simulink model "admittance"  (Simulink 8.5)
settings: Solver=ode15s  SolverMode=SingleTasking  StartTime=0.0  StopTime=0.1  RelTol=1e-3  AbsTol=1e-6
libraries: powerlib x25, powerlib_extras x6
settings Model: Creator=Dr. Lotfifard  LastModifiedBy=PC  ExtModeTrigMode=oneshot  ExtModeArmWhenConnect=off
settings DataIOCC: LimitDataPoints=off
settings OptimizationCC: BlockReduction=off  BooleanDataType=off
settings DebuggingCC: SaveWithParameterizedLinksMsg=none  SignalResolutionControl=TryResolveAllWithWarning  MultiTaskDSMMsg=warning  MultiTaskCondExecSysMsg=none  FcnCallInpInsideContextMsg=UseLocalSettings  StrictBusMsg=None
settings HardwareCC: TargetUnknown=on

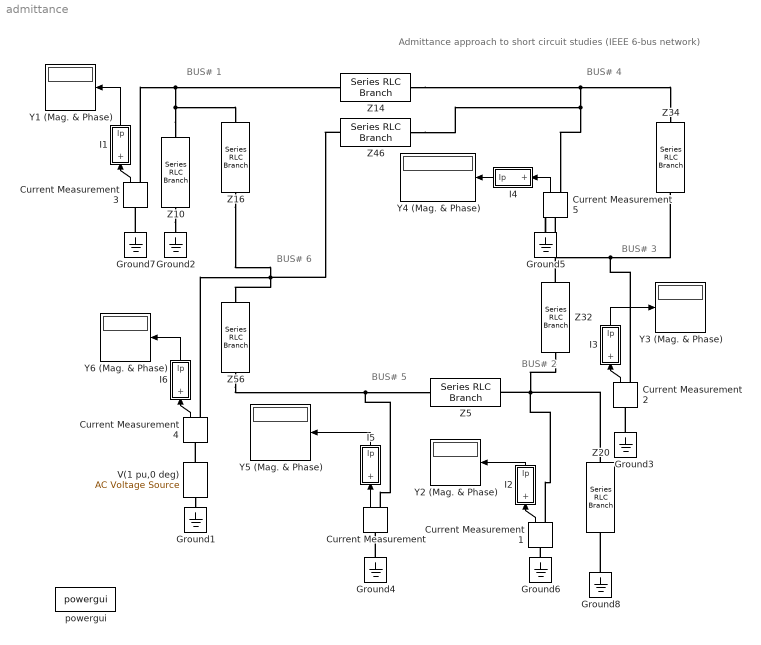
== system admittance ==
  note: Admittance approach to short circuit studies
      | (IEEE 6-bus network)
  note: BUS# 1
  note: BUS# 4
  note: BUS# 6
  note: BUS# 3
  note: BUS# 2
  note: BUS# 5
  Current Measurement{,1..5} (6 alike) : powerlib/Measurements/Current Measurement  PhasorSimulation=off  OutputType=Complex  PSBequivalent=0
  Ground{1..8} (8 alike) : powerlib/Elements/Ground  LConnTagsString=a
  I1 : Subsystem
  I2 : Subsystem
  I3 : Subsystem
  I4 : Subsystem
  I5 : Subsystem
  I6 : Subsystem
  V(1 pu,0 deg) : powerlib/Electrical Sources/AC Voltage Source  Amplitude=1  Phase=0  Frequency=60  SampleTime=0  Measurements=None
  Y1 (Mag. & Phase) : Display
  Y2 (Mag. & Phase) : Display
  Y3 (Mag. & Phase) : Display
  Y4 (Mag. & Phase) : Display
  Y5 (Mag. & Phase) : Display
  Y6 (Mag. & Phase) : Display
  Z10 : powerlib/Elements/Series RLC Branch  LConnTagsString=__new0  RConnTagsString=__new0  BranchType=RL  Resistance=0.02  Inductance=0.24/(2*pi*60)  SetiL0=off  InitialCurrent=0  Capacitance=1e-6  Setx0=off  InitialVoltage=0  Measurements=None
  Z14 : powerlib/Elements/Series RLC Branch  LConnTagsString=__new0  RConnTagsString=__new0  BranchType=RL  Resistance=0.16  Inductance=0.74/(2*pi*60)  SetiL0=off  InitialCurrent=0  Capacitance=1e-6  Setx0=off  InitialVoltage=0  Measurements=None
  Z16 : powerlib/Elements/Series RLC Branch  LConnTagsString=__new0  RConnTagsString=__new0  BranchType=RL  Resistance=0.246  Inductance=1.036/(2*pi*60)  SetiL0=off  InitialCurrent=0  Capacitance=1e-6  Setx0=off  InitialVoltage=0  Measurements=None
  Z20 : powerlib/Elements/Series RLC Branch  LConnTagsString=__new0  RConnTagsString=__new0  BranchType=RL  Resistance=0.03  Inductance=0.48/(2*pi*60)  SetiL0=off  InitialCurrent=0  Capacitance=1e-6  Setx0=off  InitialVoltage=0  Measurements=None
  Z32 : powerlib/Elements/Series RLC Branch  LConnTagsString=__new0  RConnTagsString=__new0  BranchType=RL  Resistance=1.446  Inductance=2.1/(2*pi*60)  SetiL0=off  InitialCurrent=0  Capacitance=1e-6  Setx0=off  InitialVoltage=0  Measurements=None
  Z34 : powerlib/Elements/Series RLC Branch  LConnTagsString=__new0  RConnTagsString=__new0  BranchType=RL  Resistance=0  Inductance=0.266/(2*pi*60)  SetiL0=off  InitialCurrent=0  Capacitance=1e-6  Setx0=off  InitialVoltage=0  Measurements=None
  Z46 : powerlib/Elements/Series RLC Branch  LConnTagsString=__new0  RConnTagsString=__new0  BranchType=RL  Resistance=0.194  Inductance=0.814/(2*pi*60)  SetiL0=off  InitialCurrent=0  Capacitance=1e-6  Setx0=off  InitialVoltage=0  Measurements=None
  Z5 : powerlib/Elements/Series RLC Branch  LConnTagsString=__new0  RConnTagsString=__new0  BranchType=RL  Resistance=0.564  Inductance=1.28/(2*pi*60)  SetiL0=off  InitialCurrent=0  Capacitance=1e-6  Setx0=off  InitialVoltage=0  Measurements=None
  Z56 : powerlib/Elements/Series RLC Branch  LConnTagsString=__new0  RConnTagsString=__new0  BranchType=RL  Resistance=0  Inductance=0.6/(2*pi*60)  SetiL0=off  InitialCurrent=0  Capacitance=1e-6  Setx0=off  InitialVoltage=0  Measurements=None
  powergui : powerlib/powergui  SimulationMode=Continuous  SolverType=Tustin/Backward Euler (TBE)  SampleTime=0  frequency=60  SPID=off  DisableSnubberDevices=off  DisableRonSwitches=off  DisableVfSwitches=off  SwTol=0  DisplayEquations=off  Interpol=off  methode=off  Ts=0  FunctionMessages=off  echomessages=off  HookPort=off  EnableUseOfTLC=off  x0status=blocks  frequencyindice=60  Pbase=100e6  ErrMax=1e-4  Iterations=50  UnitsV=kV  UnitsW=MW  buscounter=0  RestoreLinks=warning  ResistiveCurrentMeasurement=off  Frange=[0:2:500]  Ylog=off  Xlog=on  ShowGrid=off  save=off  variable=ZData  structure=0  ZoomFFT=on  StartTime=0.0  cycles=1  DisplayStyle=1  fundamental=60  FreqAxis=off  MaxFrequency=1000  frequencyindicesteady=1  RmsSteady=1  display=off
  wires:
  Current Measurement/1 -> I5/1(+)
  I5/1(Ip) -> Y5 (Mag. & Phase)/1
  Current Measurement1/1 -> I2/1(+)
  I2/1(Ip) -> Y2 (Mag. & Phase)/1
  Current Measurement2/1 -> I3/1(+)
  I3/1(Ip) -> Y3 (Mag. & Phase)/1
  Current Measurement3/1 -> I1/1(+)
  I1/1(Ip) -> Y1 (Mag. & Phase)/1
  Current Measurement4/1 -> I6/1(+)
  I6/1(Ip) -> Y6 (Mag. & Phase)/1
  Current Measurement5/1 -> I4/1(+)
  I4/1(Ip) -> Y4 (Mag. & Phase)/1
  connections:
  Ground4/LConn1 -- Current Measurement/LConn1
  Ground6/LConn1 -- Current Measurement1/LConn1
  Ground3/LConn1 -- Current Measurement2/LConn1
  Ground7/LConn1 -- Current Measurement3/LConn1
  V(1 pu,0 deg)/RConn1 -- Current Measurement4/LConn1
  Ground5/LConn1 -- Current Measurement5/LConn1
  Z10/RConn1 -- Ground2/LConn1
  Z10/LConn1 -- Z14/LConn1 -- Current Measurement3/RConn1 -- Z16/LConn1
  Current Measurement/RConn1 -- Z5/LConn1 -- Z56/RConn1
  Z14/RConn1 -- Z34/LConn1 -- Current Measurement5/RConn1 -- Z46/RConn1
  Z32/LConn1 -- Z34/RConn1 -- Current Measurement2/RConn1
  Z20/LConn1 -- Current Measurement1/RConn1 -- Z5/RConn1 -- Z32/RConn1
  Ground8/LConn1 -- Z20/RConn1
  V(1 pu,0 deg)/LConn1 -- Ground1/LConn1
  Z16/RConn1 -- Z56/LConn1 -- Z46/LConn1 -- Current Measurement4/RConn1

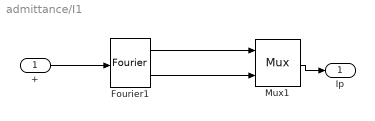
== system admittance/I1 ==
  + : Inport
  Fourier1 : powerlib_extras/Measurements/Fourier  f1=60  n=1
  Mux1 : Mux  Inputs=2
  Ip : Outport  InitialOutput=0
  wires:
  Fourier1/2 -> Mux1/2
  Fourier1/1 -> Mux1/1
  Mux1/1 -> Ip/1
  +/1 -> Fourier1/1

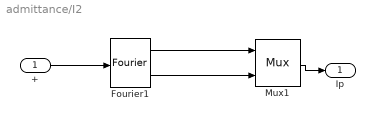
== system admittance/I2 ==
  + : Inport
  Fourier1 : powerlib_extras/Measurements/Fourier  f1=60  n=1
  Mux1 : Mux  Inputs=2
  Ip : Outport  InitialOutput=0
  wires:
  Fourier1/2 -> Mux1/2
  Fourier1/1 -> Mux1/1
  Mux1/1 -> Ip/1
  +/1 -> Fourier1/1

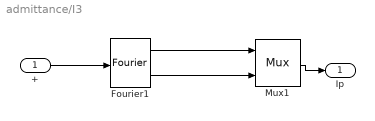
== system admittance/I3 ==
  + : Inport
  Fourier1 : powerlib_extras/Measurements/Fourier  f1=60  n=1
  Mux1 : Mux  Inputs=2
  Ip : Outport  InitialOutput=0
  wires:
  Fourier1/2 -> Mux1/2
  Fourier1/1 -> Mux1/1
  Mux1/1 -> Ip/1
  +/1 -> Fourier1/1

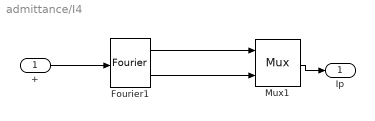
== system admittance/I4 ==
  + : Inport
  Fourier1 : powerlib_extras/Measurements/Fourier  f1=60  n=1
  Mux1 : Mux  Inputs=2
  Ip : Outport  InitialOutput=0
  wires:
  Fourier1/2 -> Mux1/2
  Fourier1/1 -> Mux1/1
  Mux1/1 -> Ip/1
  +/1 -> Fourier1/1

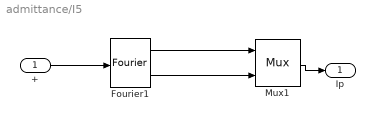
== system admittance/I5 ==
  + : Inport
  Fourier1 : powerlib_extras/Measurements/Fourier  f1=60  n=1
  Mux1 : Mux  Inputs=2
  Ip : Outport  InitialOutput=0
  wires:
  Fourier1/2 -> Mux1/2
  Fourier1/1 -> Mux1/1
  Mux1/1 -> Ip/1
  +/1 -> Fourier1/1

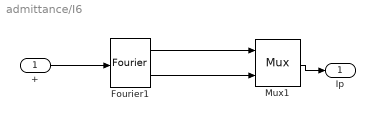
== system admittance/I6 ==
  + : Inport
  Fourier1 : powerlib_extras/Measurements/Fourier  f1=60  n=1
  Mux1 : Mux  Inputs=2
  Ip : Outport  InitialOutput=0
  wires:
  Fourier1/2 -> Mux1/2
  Fourier1/1 -> Mux1/1
  Mux1/1 -> Ip/1
  +/1 -> Fourier1/1
